simulink model "f14_dig_sf"  (Simulink 6.0)
settings: Solver=ode45  SolverMode=SingleTasking  StartTime=0.0  StopTime=1000000  FixedStep=.01  RelTol=1e-4  AbsTol=1e-6
PreLoadFcn:
  | f14dat_digital
values from neighbouring files (symbols this model uses):
  a = 2.5348    [f14dat.m]    (also in f14dat_digital.m; f14def.m)
  b = find_system('aero_atc','Type','block')    [aero_atcscript.m]    (also in f14dat.m = 64.13; f14dat_digital.m = 64.13; f14def.m = 64.13)
  deltat = pinput(23)    [aero_extkalman.m]    (also in aero_raddat.m = 1; f14dat_digital.m = 0.1)
  deltat1 = 0.01    [f14dat_digital.m]
  g = 9.81    [aero_guid_dat.m]    (also in aero_raddat.m = 32.2; f14dat.m = 32.2; f14dat_digital.m = 32.2)
  Ka = 0.6770    (= 0.677)    [f14dat.m]    (also in f14dat_digital.m; f14def.m)
  Kf = -1.7460    (= -1.746)    [f14dat.m]    (also in f14dat_digital.m; f14def.m)
  Ki = -3.8640    (= -3.864)    [f14dat.m]    (also in f14dat_digital.m; f14def.m)
  Kq = 0.8156    [f14dat.m]    (also in f14dat_digital.m; f14def.m)
  Md = -6.8847    [f14dat.m]    (also in f14dat_digital.m; f14def.m)
  Mq = -0.6571    [f14dat.m]    (also in f14dat_digital.m; f14def.m)
  Mw = -0.00592    [f14dat.m]    (also in f14dat_digital.m; f14def.m)
  Swg = 3    [f14dat.m]    (also in f14dat_digital.m; f14def.m)
  Tal = 0.3959    [f14dat.m]    (also in f14dat_digital.m; f14def.m)
  Ts = 0.1000    (= 0.1)    [f14dat.m]    (also in f14dat_digital.m; f14def.m)
  Uo = 689.4000    (= 689.4)    [f14dat.m]    (also in f14dat_digital.m; f14def.m)
  Vto = 690.4000    (= 690.4)    [f14dat.m]    (also in f14dat_digital.m; f14def.m)
  W1 = 2.9710    (= 2.971)    [f14dat.m]    (also in f14dat_digital.m; f14def.m)
  W2 = 4.1440    (= 4.144)    [f14dat.m]    (also in f14dat_digital.m; f14def.m)
  Zd = -63.9979    [f14dat.m]    (also in f14dat_digital.m; f14def.m)
  Zw = -0.6385    [f14dat.m]    (also in f14dat_digital.m; f14def.m)
undefined symbols (not defined in the file or in its folder): DiscIntNeverNeededParam
libraries: simulink x2, f14actuator x1
Description:
  | This model of the F14 is used to design a high angle of attack Digital Flight Control System.  The design works in conjunction with the GUI in F14guid.  There is documentation that goes along with this file and the
  | GUI.  The documentaiton is in the Word file "F14 Design.doc".
settings Model: Creator=The MathWorks Inc.  LastModifiedBy=batserve  ExtModeTrigMode=oneshot  ExtModeArmWhenConnect=off  ExtModeAutoUpdateStatusClock=off
settings DataIOCC: ExternalInput=[]  InitialState=[]  LimitDataPoints=off  SaveOutput=off  SaveTime=off  SignalLoggingName=logsOut
settings OptimizationCC: BlockReduction=off  BooleanDataType=off
settings DebuggingCC: CheckExecutionContextPreStartOutputMsg=on  CheckExecutionContextRuntimeOutputMsg=on  SolverPrmCheckMsg=none  IntegerOverflowMsg=none
settings HardwareCC: TargetUnknown=on
settings RTWCC: GenCodeOnly=on  TemplateMakefile=grt_vc.tmf

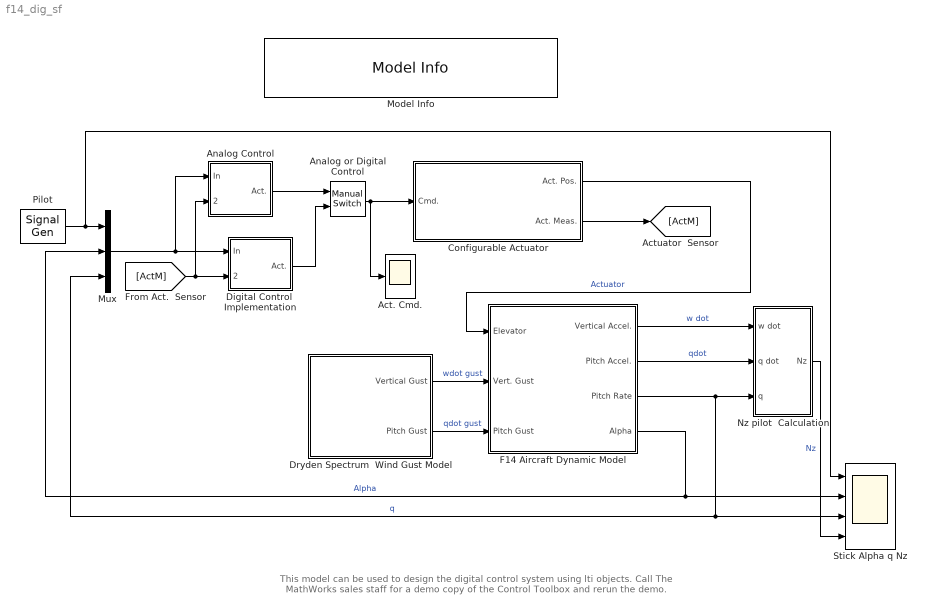
== system f14_dig_sf ==
  note: This model can be used to design the digital
      | control system using lti objects.
      | Call The MathWorks sales staff for a demo
      | copy of the Control Toolbox and rerun the demo.
  Act. Cmd. : Scope
      settings: TickLabels=on  TimeRange=15  YMin=-2.5  YMax=2.5  DataFormat=Array
  Analog Control : Subsystem  PropExecContextAcrossSSBoundary=on
  Analog or Digital Control : simulink/Signal Routing/Manual Switch  sw=0  action=0
  Configurable Actuator : Subsystem  BlockChoice=Linear Actuator Subsystem  PropExecContextAcrossSSBoundary=on
      settings: MemberBlocks=Linear Actuator Subsystem,Non-Linear Actuator Subsystem
      settings: TemplateBlock=|
      | f14actuator/Configurable
      | Actuator
  Digital Control  Implementation : Subsystem  PropExecContextAcrossSSBoundary=on
  Dryden Spectrum  Wind Gust Model : Subsystem  PropExecContextAcrossSSBoundary=on
      mask Display: image(weatherrgb)
  F14 Aircraft Dynamic Model : Subsystem  PropExecContextAcrossSSBoundary=on
      mask Display: image(rgb)
  Model Info : simulink/Model-Wide Utilities/Model Info  InitialBlockCM=none  BlockCM=none  Frame=off  DisplayStringWithTags="F14 High Angle of Attack  Digital Flight Control System"  HorizontalTextAlignment=Center  LeftAlignmentValue=0.5  SourceBlockDiagram=f14_dig_sf  TagMaxNumber=20
  Mux : Mux  Inputs=3
  Nz pilot  Calculation : Subsystem  PropExecContextAcrossSSBoundary=on
  Pilot : SignalGenerator  WaveForm=square  Frequency=0.500000  Units=rad/sec
  Stick Alpha q Nz : Scope  NumInputPorts=4
      settings: TickLabels=on  TimeRange=15  YMin=-1~-1.5~-3~-15  YMax=1~1.5~3~15  DataFormat=Array
  wires:
  Dryden Spectrum  Wind Gust Model/1(Vertical Gust) -> F14 Aircraft Dynamic Model/2(Vert. Gust)  "wdot gust"
  Dryden Spectrum  Wind Gust Model/2(Pitch Gust) -> F14 Aircraft Dynamic Model/3(Pitch Gust)  "qdot gust"
  Pilot/1 -> Mux/1, Stick Alpha q Nz/1
  F14 Aircraft Dynamic Model/1(Vertical Accel.) -> Nz pilot  Calculation/1(w dot)  "w dot"
  F14 Aircraft Dynamic Model/2(Pitch Accel.) -> Nz pilot  Calculation/2(q dot)  "qdot"
  F14 Aircraft Dynamic Model/3(Pitch Rate) -> Nz pilot  Calculation/3(q), Stick Alpha q Nz/3, Mux/3  "q"
  F14 Aircraft Dynamic Model/4(Alpha) -> Mux/2, Stick Alpha q Nz/2  "Alpha"
  Nz pilot  Calculation/1(Nz) -> Stick Alpha q Nz/4  "Nz"
  Analog or Digital Control/1 -> Configurable Actuator/1(Cmd.), Act. Cmd./1
  Analog Control/1(Act.) -> Analog or Digital Control/1
  Digital Control  Implementation/1(Act.) -> Analog or Digital Control/2
  Mux/1 -> Analog Control/1(In), Digital Control  Implementation/1(In)
  [ActM] -> Analog Control/2(Actuator Pos.), Digital Control  Implementation/2(Actuator Pos.)
  Configurable Actuator/2(Act. Meas.) -> [ActM]
  Configurable Actuator/1(Act. Pos.) -> F14 Aircraft Dynamic Model/1(Elevator)  "Actuator"

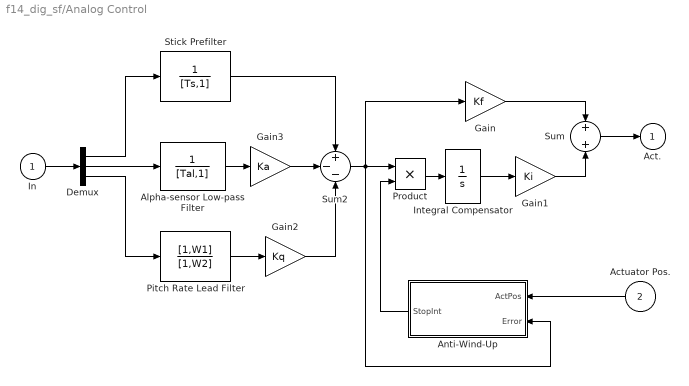
== system f14_dig_sf/Analog Control ==
  In : Inport  Port=1  LatchInput=off
  Actuator Pos. : Inport  Orientation=left  Port=2  LatchInput=off
  Alpha-sensor Low-pass Filter : TransferFcn  Denominator=[Tal,1]
  Anti-Wind-Up : Stateflow chart  Orientation=left  PropExecContextAcrossSSBoundary=on
  Demux : Demux  Outputs=3
  Gain : Gain  Gain=Kf  SaturateOnIntegerOverflow=on
  Gain1 : Gain  Gain=Ki  SaturateOnIntegerOverflow=on
  Gain2 : Gain  Gain=Kq  SaturateOnIntegerOverflow=on
  Gain3 : Gain  Gain=Ka  SaturateOnIntegerOverflow=on
  Integral Compensator : TransferFcn  Denominator=[1,0]
  Pitch Rate Lead Filter : TransferFcn  Numerator=[1,W1]  Denominator=[1,W2]
  Product : Product  SaturateOnIntegerOverflow=on  RndMeth=Zero  InputSameDT=on
  Stick Prefilter : TransferFcn  Denominator=[Ts,1]
  Sum : Sum  Inputs=2  SaturateOnIntegerOverflow=on  InputSameDT=on
  Sum2 : Sum  Inputs=+--  SaturateOnIntegerOverflow=on  InputSameDT=on
  Act. : Outport  InitialOutput=0
  wires:
  Sum/1 -> Act./1
  In/1 -> Demux/1
  Alpha-sensor Low-pass Filter/1 -> Gain3/1
  Gain2/1 -> Sum2/3
  Stick Prefilter/1 -> Sum2/1
  Pitch Rate Lead Filter/1 -> Gain2/1
  Demux/1 -> Stick Prefilter/1
  Demux/2 -> Alpha-sensor Low-pass Filter/1
  Demux/3 -> Pitch Rate Lead Filter/1
  Gain3/1 -> Sum2/2
  Gain/1 -> Sum/1
  Actuator Pos./1 -> Anti-Wind-Up/1(ActPos)
  Sum2/1 -> Gain/1, Product/1, Anti-Wind-Up/2(Error)
  Gain1/1 -> Sum/2
  Integral Compensator/1 -> Gain1/1
  Product/1 -> Integral Compensator/1
  Anti-Wind-Up/1(StopInt) -> Product/2

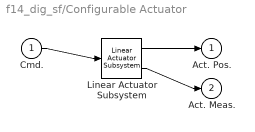
== system f14_dig_sf/Configurable Actuator ==
  Cmd. : Inport  Port=1  LatchInput=off
  Linear Actuator Subsystem : f14actuator/Linear Actuator Subsystem
  Act. Pos. : Outport
  Act. Meas. : Outport  Port=2
  wires:
  Cmd./1 -> Linear Actuator Subsystem/1
  Linear Actuator Subsystem/1 -> Act. Pos./1
  Linear Actuator Subsystem/2 -> Act. Meas./1

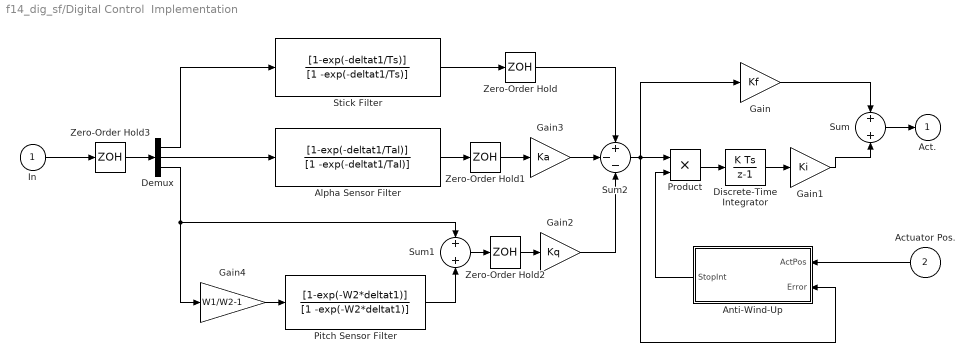
== system f14_dig_sf/Digital Control  Implementation ==
  In : Inport  Port=1  LatchInput=off
  Actuator Pos. : Inport  Orientation=left  Port=2  LatchInput=off
  Alpha Sensor Filter : DiscreteTransferFcn  Numerator=[1-exp(-deltat1/Tal)]  Denominator=[1 -exp(-deltat1/Tal)]  SampleTime=deltat1
  Anti-Wind-Up : Stateflow chart  Orientation=left  PropExecContextAcrossSSBoundary=on
  Demux : Demux  Outputs=3
  Discrete-Time Integrator : DiscreteIntegrator  SampleTime=deltat  ICPrevOutput=DiscIntNeverNeededParam  ICPrevScaledInput=DiscIntNeverNeededParam
  Gain : Gain  Gain=Kf  SaturateOnIntegerOverflow=on
  Gain1 : Gain  Gain=Ki  SaturateOnIntegerOverflow=on
  Gain2 : Gain  Gain=Kq  SaturateOnIntegerOverflow=on
  Gain3 : Gain  Gain=Ka  SaturateOnIntegerOverflow=on
  Gain4 : Gain  Gain=W1/W2-1  SaturateOnIntegerOverflow=on
  Pitch Sensor Filter : DiscreteTransferFcn  Numerator=[1-exp(-W2*deltat1)]  Denominator=[1 -exp(-W2*deltat1)]  SampleTime=deltat1
  Product : Product  SaturateOnIntegerOverflow=on  RndMeth=Zero  InputSameDT=on
  Stick Filter : DiscreteTransferFcn  Numerator=[1-exp(-deltat1/Ts)]  Denominator=[1 -exp(-deltat1/Ts)]  SampleTime=deltat1
  Sum : Sum  Inputs=2  SaturateOnIntegerOverflow=on  InputSameDT=on
  Sum1 : Sum  Inputs=2  SaturateOnIntegerOverflow=on  InputSameDT=on
  Sum2 : Sum  Inputs=+--  SaturateOnIntegerOverflow=on  InputSameDT=on
  Zero-Order Hold : ZeroOrderHold  SampleTime=deltat
  Zero-Order Hold1 : ZeroOrderHold  SampleTime=deltat
  Zero-Order Hold2 : ZeroOrderHold  SampleTime=deltat
  Zero-Order Hold3 : ZeroOrderHold  SampleTime=deltat1
  Act. : Outport  InitialOutput=0
  wires:
  Gain2/1 -> Sum2/3
  Sum/1 -> Act./1
  Sum2/1 -> Gain/1, Anti-Wind-Up/2(Error), Product/1
  Demux/2 -> Alpha Sensor Filter/1
  Demux/3 -> Sum1/1, Gain4/1
  Demux/1 -> Stick Filter/1
  Stick Filter/1 -> Zero-Order Hold/1
  Zero-Order Hold/1 -> Sum2/1
  Alpha Sensor Filter/1 -> Zero-Order Hold1/1
  Zero-Order Hold1/1 -> Gain3/1
  Sum1/1 -> Zero-Order Hold2/1
  In/1 -> Zero-Order Hold3/1
  Zero-Order Hold3/1 -> Demux/1
  Pitch Sensor Filter/1 -> Sum1/2
  Gain4/1 -> Pitch Sensor Filter/1
  Zero-Order Hold2/1 -> Gain2/1
  Gain3/1 -> Sum2/2
  Gain/1 -> Sum/1
  Gain1/1 -> Sum/2
  Actuator Pos./1 -> Anti-Wind-Up/1(ActPos)
  Product/1 -> Discrete-Time Integrator/1
  Discrete-Time Integrator/1 -> Gain1/1
  Anti-Wind-Up/1(StopInt) -> Product/2

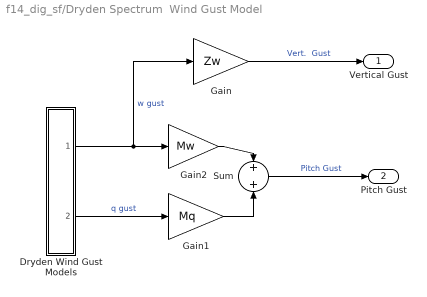
== system f14_dig_sf/Dryden Spectrum  Wind Gust Model ==
  Dryden Wind Gust Models : Subsystem  PropExecContextAcrossSSBoundary=on
  Gain : Gain  Gain=Zw  SaturateOnIntegerOverflow=on
  Gain1 : Gain  Gain=Mq  SaturateOnIntegerOverflow=on
  Gain2 : Gain  Gain=Mw  SaturateOnIntegerOverflow=on
  Sum : Sum  SaturateOnIntegerOverflow=on  InputSameDT=on
  Vertical Gust : Outport
  Pitch Gust : Outport  Port=2
  wires:
  Dryden Wind Gust Models/2(Qg) -> Gain1/1  "q gust"
  Dryden Wind Gust Models/1(Wg) -> Gain2/1, Gain/1  "w gust"
  Gain2/1 -> Sum/1
  Gain1/1 -> Sum/2
  Gain/1 -> Vertical Gust/1  "Vert.  Gust"
  Sum/1 -> Pitch Gust/1  "Pitch Gust"

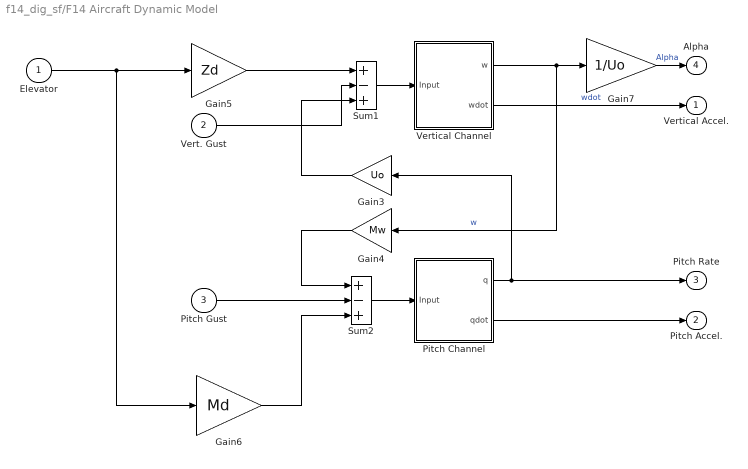
== system f14_dig_sf/F14 Aircraft Dynamic Model ==
  Elevator : Inport  Port=1  LatchInput=off
  Vert. Gust : Inport  Port=2  LatchInput=off
  Pitch Gust : Inport  Port=3  LatchInput=off
  Gain3 : Gain  Orientation=left  Gain=Uo  SaturateOnIntegerOverflow=on
  Gain4 : Gain  Orientation=left  Gain=Mw  SaturateOnIntegerOverflow=on
  Gain5 : Gain  Gain=Zd  SaturateOnIntegerOverflow=on
  Gain6 : Gain  Gain=Md  SaturateOnIntegerOverflow=on
  Gain7 : Gain  Gain=1/Uo  SaturateOnIntegerOverflow=on
  Pitch Channel : Subsystem  PropExecContextAcrossSSBoundary=on
  Sum1 : Sum  Inputs=+-+  SaturateOnIntegerOverflow=on  InputSameDT=on
  Sum2 : Sum  Inputs=+-+  SaturateOnIntegerOverflow=on  InputSameDT=on
  Vertical Channel : Subsystem  PropExecContextAcrossSSBoundary=on
  Vertical Accel. : Outport  InitialOutput=0
  Pitch Accel. : Outport  Port=2  InitialOutput=0
  Pitch Rate : Outport  Port=3  InitialOutput=0
  Alpha : Outport  Port=4  InitialOutput=0
  wires:
  Pitch Channel/2(qdot) -> Pitch Accel./1
  Pitch Channel/1(q) -> Pitch Rate/1, Gain3/1
  Vertical Channel/2(wdot) -> Vertical Accel./1  "wdot"
  Vertical Channel/1(w) -> Gain4/1, Gain7/1  "w"
  Sum1/1 -> Vertical Channel/1(Input)
  Gain6/1 -> Sum2/3
  Gain5/1 -> Sum1/1
  Gain3/1 -> Sum1/3
  Pitch Gust/1 -> Sum2/2
  Sum2/1 -> Pitch Channel/1(Input)
  Gain4/1 -> Sum2/1
  Vert. Gust/1 -> Sum1/2
  Elevator/1 -> Gain5/1, Gain6/1
  Gain7/1 -> Alpha/1  "Alpha"

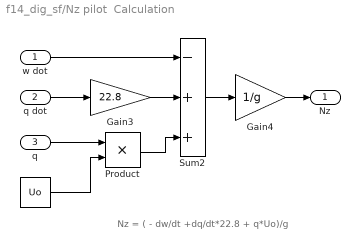
== system f14_dig_sf/Nz pilot  Calculation ==
  note: Nz = ( - dw/dt +dq/dt*22.8 + q*Uo)/g
  w dot : Inport  Port=1  LatchInput=off
  q dot : Inport  Port=2  LatchInput=off
  q : Inport  Port=3  LatchInput=off
  " " : Constant  Value=Uo
  Gain3 : Gain  Gain=22.8  SaturateOnIntegerOverflow=on
  Gain4 : Gain  Gain=1/g  SaturateOnIntegerOverflow=on
  Product : Product  SaturateOnIntegerOverflow=on  RndMeth=Zero  InputSameDT=on
  Sum2 : Sum  Inputs=-++  SaturateOnIntegerOverflow=on  InputSameDT=on
  Nz : Outport  InitialOutput=0
  wires:
  Sum2/1 -> Gain4/1
  w dot/1 -> Sum2/1
  Gain4/1 -> Nz/1
  q dot/1 -> Gain3/1
  Gain3/1 -> Sum2/2
  Product/1 -> Sum2/3
  q/1 -> Product/1
  " "/1 -> Product/2

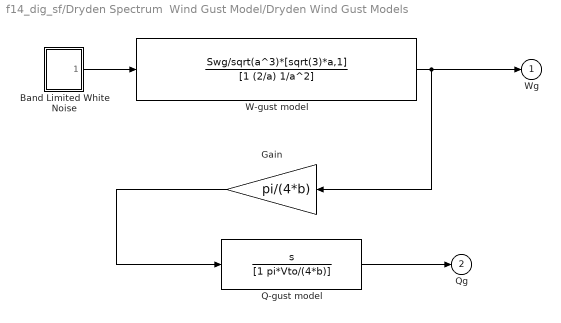
== system f14_dig_sf/Dryden Spectrum  Wind Gust Model/Dryden Wind Gust Models ==
  Band Limited White Noise : Subsystem  PropExecContextAcrossSSBoundary=on  mask(Continuous White Noise.){Cov=10, Ts=0.1, seed=23341}
      mask prompts: Cov "Noise Variance:"; Ts "Sample Time:"
      mask help:
      | White noise for continuous (s-domain) systems.
      | Band-limited using zero-order-hold.
      mask init:
      | r = rand(1,12); r2 = [r(1),r;r,r(12)]; t =[1:13;1:13];
      mask Help: Implemented using white noise into Zero Order Hold block. For faster simulation set sample time to highest value possible but in accordance with the fastest dynamics of system.
      mask Display: plot(t(:),r2(:))
  Gain : Gain  Orientation=left  Gain=pi/(4*b)  SaturateOnIntegerOverflow=on
  Q-gust model : TransferFcn  Numerator=[1 0]  Denominator=[1 pi*Vto/(4*b)]
  W-gust model : TransferFcn  Numerator=Swg/sqrt(a^3)*[sqrt(3)*a,1]  Denominator=[1 (2/a) 1/a^2]
  Wg : Outport  InitialOutput=0
  Qg : Outport  Port=2  InitialOutput=0
  wires:
  W-gust model/1 -> Gain/1, Wg/1
  Band Limited White Noise/1(out_1) -> W-gust model/1
  Gain/1 -> Q-gust model/1
  Q-gust model/1 -> Qg/1

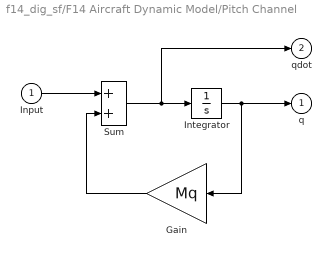
== system f14_dig_sf/F14 Aircraft Dynamic Model/Pitch Channel ==
  Input : Inport  Port=1  LatchInput=off
  Gain : Gain  Orientation=left  Gain=Mq  SaturateOnIntegerOverflow=on
  Integrator : Integrator
  Sum : Sum  SaturateOnIntegerOverflow=on  InputSameDT=on
  q : Outport  InitialOutput=0
  qdot : Outport  Port=2  InitialOutput=0
  wires:
  Input/1 -> Sum/1
  Gain/1 -> Sum/2
  Integrator/1 -> q/1, Gain/1
  Sum/1 -> Integrator/1, qdot/1

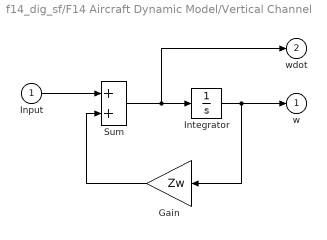
== system f14_dig_sf/F14 Aircraft Dynamic Model/Vertical Channel ==
  Input : Inport  Port=1  LatchInput=off
  Gain : Gain  Orientation=left  Gain=Zw  SaturateOnIntegerOverflow=on
  Integrator : Integrator
  Sum : Sum  SaturateOnIntegerOverflow=on  InputSameDT=on
  w : Outport  InitialOutput=0
  wdot : Outport  Port=2  InitialOutput=0
  wires:
  Sum/1 -> wdot/1, Integrator/1
  Integrator/1 -> Gain/1, w/1
  Gain/1 -> Sum/2
  Input/1 -> Sum/1

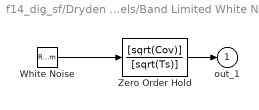
== system f14_dig_sf/Dryden Spectrum  Wind Gust Model/Dryden Wind Gust Models/Band Limited White Noise ==
  White Noise : RandomNumber  Seed=seed  SampleTime=Ts
  Zero Order Hold : DiscreteTransferFcn  Numerator=[sqrt(Cov)]  Denominator=[sqrt(Ts)]  SampleTime=Ts
  out_1 : Outport  InitialOutput=0
  wires:
  Zero Order Hold/1 -> out_1/1
  White Noise/1 -> Zero Order Hold/1

== stateflow chart Analog Control/Anti-Wind-Up ==
  state Integrate
    en:StopInt=1;
  state Stop_Integrating
    en: StopInt=0;
  (default) -> Integrate
  Integrate -> Stop_Integrating : [abs(ActPos)>Sat  &  ActPos*Error >0]
  Stop_Integrating -> Integrate : [abs(ActPos)<Sat ]
  data: ActPos input double; Error input double; StopInt output double; Sat constant double =0.785398

== stateflow chart Digital Control Implementation/Anti-Wind-Up ==
  state Integrate
    en:StopInt=1;
  state Stop_Integrating
    en: StopInt=0;
  (default) -> Integrate
  Integrate -> Stop_Integrating : [abs(ActPos)>Sat  &  ActPos*Error >0]
  Stop_Integrating -> Integrate : [abs(ActPos)<Sat ]
  data: ActPos input double; Error input double; StopInt output double; Sat constant double =0.785398
